simulink model "eliminationOfInversedThermocline"  (R2016b)
settings: Solver=ode45  StartTime=0.0  StopTime=2*3600  MaxStep=300  RelTol=1e-3  EnableMultiTasking=on
libraries: carnot x15
settings Model: Creator=drhf  LastModifiedBy=drhf
settings DataIOCC: LimitDataPoints=on  SaveFormat=Array  SignalLoggingSaveFormat=ModelDataLogs
settings OptimizationCC: ExpressionDepthLimit=2147483647  LifeSpan=inf
settings DebuggingCC: UnderspecifiedInitializationDetection=Classic  MergeDetectMultiDrivingBlocksExec=none  SolverPrmCheckMsg=warning  FcnCallInpInsideContextMsg=warning  StateNameClashWarn=warning  SFUnexpectedBacktrackingDiag=warning  SFNoUnconditionalDefaultTransitionDiag=warning  SFExecutionAtInitializationDiag=none
settings HardwareCC: ProdBitPerPointer=32  ProdBitPerSizeT=32  ProdBitPerPtrDiffT=32  ProdLargestAtomicFloat=None  ProdIntDivRoundTo=Undefined  ProdEndianess=Unspecified  ProdWordSize=32  ProdHWDeviceType=32-bit Generic
settings ModelReferenceCC: PropagateSignalLabelsOutOfModel=off
settings GRTTargetCC: TargetLangStandard=C89/C90 (ANSI)  GeneratePreprocessorConditionals=Disable all  CombineOutputUpdateFcns=off  GRTInterface=on
settings ConfigComp: CovMetricSettings=dw  CovHtmlReporting=on  CovSaveCumulativeToWorkspaceVar=on  CovSaveSingleToWorkspaceVar=on  CovExternalEMLEnable=off

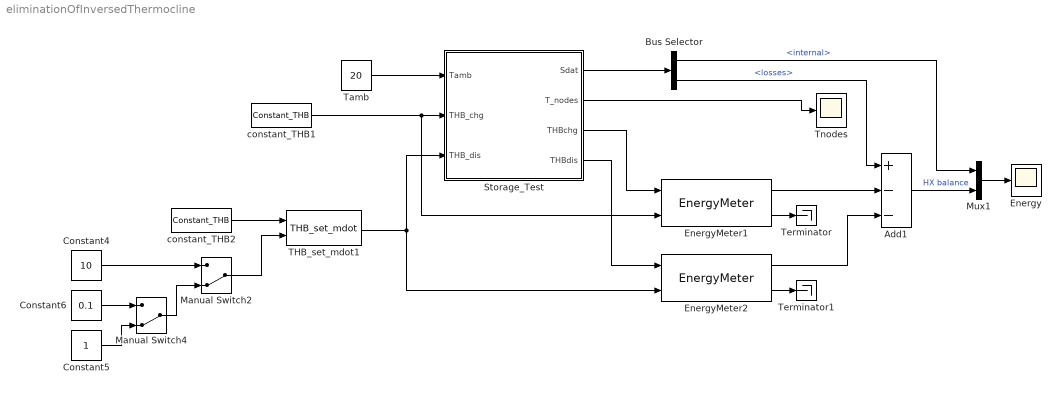
== system eliminationOfInversedThermocline ==
  Add1 : Sum  Inputs=+--
  Bus Selector : BusSelector  OutputSignals=energy.internal,energy.losses
  Constant4 : Constant  Value=10
  Constant5 : Constant
  Constant6 : Constant  Value=0.1
  Energy : Scope
  EnergyMeter1 : carnot/Control/EnergyMeter
  EnergyMeter2 : carnot/Control/EnergyMeter
  Manual Switch2 : ManualSwitch  CurrentSetting=0
  Manual Switch4 : ManualSwitch  CurrentSetting=0
  Mux1 : Mux  Inputs=2
  Storage_Test : Subsystem  mask(Multiport Storage){uloss=0, ubot=0, utop=0, cond=0, t0=10, volume=3, dia=1, pos=standing cylinder, nconnect=2, nodes=100, mpoints=5}
      mask prompts: uloss "Heat loss coefficient cylinder wall in W/(m²K)"; ubot "Heat loss coefficient bottom in W/(m²K)"; utop "Heat loss coefficient top cover in W/(m²K)"; cond "Effective vertical conductivity in W/(m*K)"; t0 "Initial temperature (vector or scalar) in °C"; volume "Volume in m³"; dia "Diameter in m"; pos "Position"; nconnect "Number of connections"; nodes "Number of nodes"; mpoints "Number of measurement points"
      mask help:
      | The volmue of the cylindrical storage is divided in a number "nodes" of horizontal slices (1xN-node model). For each node the energy balance equation is solved.
      | Look under mask to set the ports types and properties.
      mask init:
      | [standing, dh, height, mpts, tini] ...
      |     = CarnotCallbacks_StorageTypeN(pos, volume, dia, nodes, mpoints, t0);
      mask Help: web(fullfile(path_carnot('help'),'storage_multiport.html'),'-helpbrowser')
      mask TypeOptions pos: lying cylinder | standing cylinder
      mask Display: plot(10,10,90,100,[40,40,45,55,60,60,55,45,40],[84,36,30,30,36,84,90,90,84],[40,35],[77,77],[64,60],[77,77],[40,35],[42,42],[64,60],[42,42])
  THB_set_mdot1 : carnot/Source/Simple/THB_set_mdot
  Tamb : Constant  Value=20
  Terminator : Terminator
  Terminator1 : Terminator
  Tnodes : Scope
  constant_THB1 : carnot/Source/Simple/Constant_THB  t=55  mdot=0*100/3600  p=1e5  mID=Full Pressure Drop with Static Height  fluid=Water  mix=0  mix2=0  mix3=0  dia=0.02  hgt=0
  constant_THB2 : carnot/Source/Simple/Constant_THB  t=60  mdot=100/3600  p=1e5  mID=Full Pressure Drop with Static Height  fluid=Water  mix=0  mix2=0  mix3=0  dia=0.02  hgt=0
  wires:
  Bus Selector/1 -> Mux1/1  "<internal>"
  Tamb/1 -> Storage_Test/1(Tamb)
  constant_THB1/1 -> EnergyMeter1/2, Storage_Test/2(THB_chg)
  THB_set_mdot1/1 -> Storage_Test/3(THB_dis), EnergyMeter2/2
  Storage_Test/1(Sdat) -> Bus Selector/1
  Storage_Test/2(T_nodes) -> Tnodes/1
  Storage_Test/3(THBchg) -> EnergyMeter1/1
  Storage_Test/4(THBdis) -> EnergyMeter2/1
  Mux1/1 -> Energy/1
  constant_THB2/1 -> THB_set_mdot1/1
  Manual Switch2/1 -> THB_set_mdot1/2
  Add1/1 -> Mux1/2  "HX balance"
  EnergyMeter2/1 -> Add1/3
  EnergyMeter1/1 -> Add1/2
  Bus Selector/2 -> Add1/1  "<losses>"
  Constant4/1 -> Manual Switch2/1
  Constant6/1 -> Manual Switch4/1
  Manual Switch4/1 -> Manual Switch2/2
  Constant5/1 -> Manual Switch4/2
  EnergyMeter1/2 -> Terminator/1
  EnergyMeter2/2 -> Terminator1/1

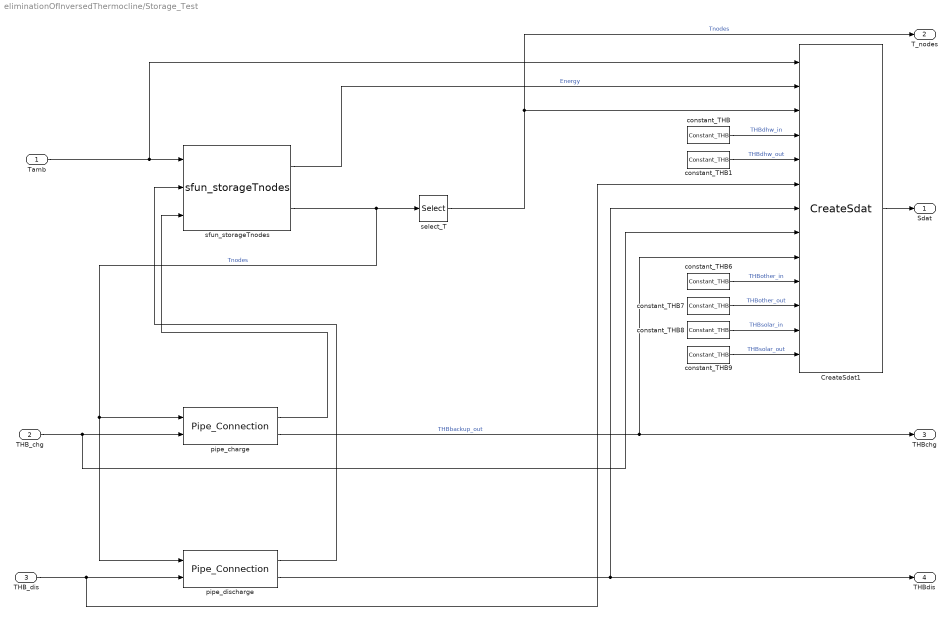
== system eliminationOfInversedThermocline/Storage_Test ==
  Tamb : Inport
  THB_chg : Inport  Port=2
  THB_dis : Inport  Port=3
  CreateSdat1 : carnot/Basic/Thermal_Models/CreateSdat  volume=0.1
  constant_THB{,1,6..9} (6 alike) : carnot/Source/Simple/Constant_THB  t=20  mdot=0  p=1e5  mID=No Pressure Drop  fluid=Water  mix=0  mix2=0  mix3=0  dia=0.02  hgt=0
  pipe_charge : carnot/Storage/Thermal/Storage_Ports/Pipe_Connection  h_in=1  h_out=0  hgt=height  dia=dia  height=-3.8197  nodes=nodes
  pipe_discharge : carnot/Storage/Thermal/Storage_Ports/Pipe_Connection  h_in=0  h_out=1  hgt=height  dia=dia  height=3.8197  nodes=nodes
  select_T : Selector  InputPortWidth=nodes  IndexOptions=Index vector (dialog)  Indices=mpts  OutputSizes=1
  sfun_storageTnodes : carnot/Basic/Thermal_Models/sfun_storageTnodes  uloss=uloss  ubot=utop  utop=ubot  cond=cond  volume=volume  dia=dia  standing=standing  tini=tini  nodes=nodes  nconnect=nconnect  elimthermocline=2  condinvtc=1e5
  Sdat : Outport
  T_nodes : Outport  Port=2
  THBchg : Outport  Port=3
  THBdis : Outport  Port=4
  wires:
  pipe_charge/1 -> sfun_storageTnodes/3
  pipe_charge/2 -> CreateSdat1/9, THBchg/1  "THBbackup_out"
  THB_chg/1 -> CreateSdat1/8, pipe_charge/2
  sfun_storageTnodes/2 -> pipe_discharge/1, pipe_charge/1, select_T/1  "Tnodes"
  sfun_storageTnodes/1 -> CreateSdat1/2  "Energy"
  select_T/1 -> T_nodes/1, CreateSdat1/3  "Tnodes"
  pipe_discharge/1 -> sfun_storageTnodes/2
  pipe_discharge/2 -> CreateSdat1/7, THBdis/1
  THB_dis/1 -> CreateSdat1/6, pipe_discharge/2
  Tamb/1 -> CreateSdat1/1, sfun_storageTnodes/1
  constant_THB/1 -> CreateSdat1/4  "THBdhw_in"
  constant_THB1/1 -> CreateSdat1/5  "THBdhw_out"
  constant_THB6/1 -> CreateSdat1/10  "THBother_in"
  constant_THB7/1 -> CreateSdat1/11  "THBother_out"
  constant_THB8/1 -> CreateSdat1/12  "THBsolar_in"
  constant_THB9/1 -> CreateSdat1/13  "THBsolar_out"
  CreateSdat1/1 -> Sdat/1
